simulink model "statefdbk_2015"  (R2015b)
settings: Solver=VariableStepAuto  StartTime=0.0  StopTime=10.0  RelTol=1e-3
values from neighbouring files (symbols this model uses):
  A1 = A-B*K-L*C    [Exe1-old.m]    (also in Exe1.m)
  B1 = L    [Exe1-old.m]    (also in Exe1.m)
  C1 = -K    [Exe1-old.m]    (also in Exe1.m)
  D2 = [0 0]    [Exe1-old.m]    (also in Exe1.m)
  x0 = [0.1 0 0 0 0]'    [Exe1-old.m]    (also in Exe1.m)
undefined symbols (not defined in the file or in its folder): A, B, C, D
settings Model: Creator=CMNO  LastModifiedBy=CMNO

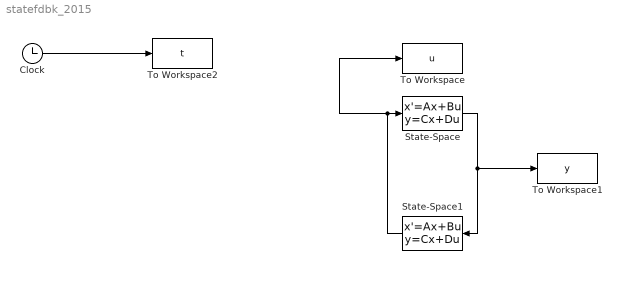
== system statefdbk_2015 ==
  Clock : Clock
  State-Space : StateSpace  A=A  B=B  C=C  D=D  X0=x0
  State-Space1 : StateSpace  A=A1  B=B1  C=C1  D=D2  X0=0
  To Workspace : ToWorkspace  VariableName=u  SaveFormat=Timeseries  SampleTime=-1
  To Workspace1 : ToWorkspace  VariableName=y  SaveFormat=Timeseries  SampleTime=-1
  To Workspace2 : ToWorkspace  VariableName=t  SaveFormat=Timeseries  SampleTime=-1
  wires:
  State-Space/1 -> To Workspace1/1, State-Space1/1
  State-Space1/1 -> To Workspace/1, State-Space/1
  Clock/1 -> To Workspace2/1
